simulink model "cannon2"  (R2025b)
settings: Solver=VariableStepAuto  StartTime=0.0  StopTime=20.0  RelTol=1e-3
settings Model: Creator=Administrator  LastModifiedBy=Administrator

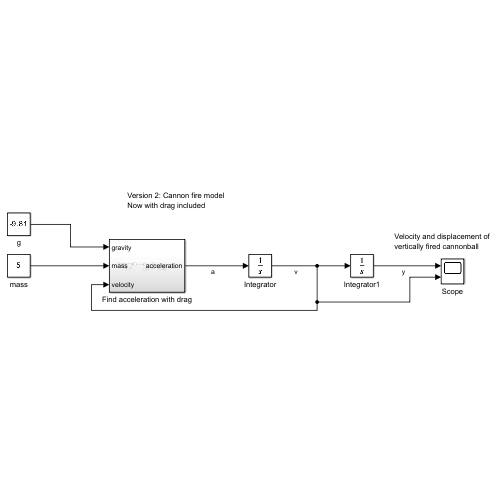
[thumbnail: Simulink's stored preview of the top-level diagram]
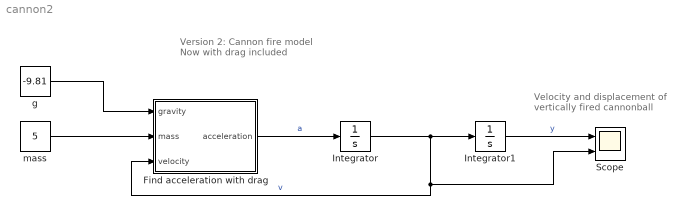
== system cannon2 ==
  note: Velocity and displacement of
      | vertically fired cannonball
  note: Version 2: Cannon fire model
      | Now with drag included
  Find acceleration with drag : Subsystem
  Integrator : Integrator  InitialCondition=100
  Integrator1 : Integrator
  Scope : Scope  NumInputPorts=2
      settings: ActiveDisplayYMinimum=-1044.7875111486396  ActiveDisplayYMaximum=415.1165915826972
  g : Constant  Value=-9.81
  mass : Constant  Value=5
  wires:
  g/1 -> Find acceleration with drag/1(gravity)
  Integrator/1 -> Scope/2, Find acceleration with drag/3(velocity), Integrator1/1  "v"
  Integrator1/1 -> Scope/1  "y"
  mass/1 -> Find acceleration with drag/2(mass)
  Find acceleration with drag/1(acceleration) -> Integrator/1  "a"

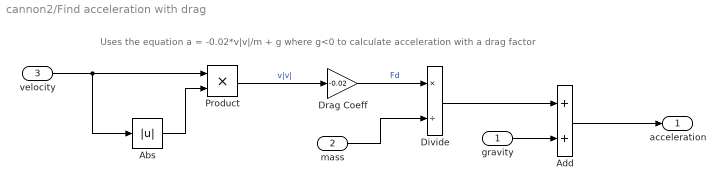
== system cannon2/Find acceleration with drag ==
  note: Uses the equation a = -0.02*v|v|/m + g where g<0 to calculate acceleration with a drag factor
  gravity : Inport
  mass : Inport  Port=2
  velocity : Inport  Port=3
  Abs : Abs  SaturateOnIntegerOverflow=off
  Add : Sum
  Divide : Product  Inputs=*/
  Drag Coeff : Gain  Gain=-0.02
  Product : Product
  acceleration : Outport
  wires:
  velocity/1 -> Abs/1, Product/1
  Abs/1 -> Product/2
  Product/1 -> Drag Coeff/1  "v|v|"
  Drag Coeff/1 -> Divide/1  "Fd"
  mass/1 -> Divide/2
  Divide/1 -> Add/1
  gravity/1 -> Add/2
  Add/1 -> acceleration/1
